simulink model "BugE_v0_40_MAS"  (R2015b)
settings: Solver=FixedStepDiscrete  StartTime=0.0  StopTime=inf  FixedStep=sample_time  RelTol=1e-3
values from neighbouring files (symbols this model uses):
  AB_diode_dV = 0.9    [main_sync.m]
  air_density = 1.225    [main_sync.m]
  bus_charger_Pmax = 1000    [main_sync.m]
  bus_load_Pmax_abs = 500    [main_sync.m]
  capInitVolt = capVmax*sqrt(capInitSoC)    [main_sync.m]
  cyc_kph = [cyc_kph(:,1), cyc_kph(:,2)*speed_max_limit/speed_max]    [main_sync.m]
  cyc_repeat = 0    [main_sync.m]
  ess1_init_soc = 1    [main_sync.m]
  ess1_soh = 1    [main_sync.m]
  ess2_init_soc = 1    [main_sync.m]
  ess2_soh = 1    [main_sync.m]
  ess3_init_soc = 1    [main_sync.m]
  ess3_soh = 1    [main_sync.m]
  ess4_init_soc = 1    [main_sync.m]
  ess4_soh = 1    [main_sync.m]
  ess5_init_soc = 1    [main_sync.m]
  ess5_soh = 1    [main_sync.m]
  gear_ratio = 6    [main_sync.m]
  loadpower = rawcsv(:,2)    [main_sync.m]
  loadtime = rawcsv(:,1)    [main_sync.m]
  lockSOCs = 0    [main_sync.m]
  max_brk_torque = 300    [main_sync.m]
  no_wheels = 3    [main_sync.m]
  period2 = max(loadtime)    [main_sync.m]
  PV_Pmax = 100    [main_sync.m]
  sample_time = 0.01    [main_sync.m]
  startup_seq_step_delay = 0.2    [main_sync.m]
  stop_option = 0    [main_sync.m]
  use_drive_cycle = 1    [main_sync.m]
  use_real_subs_loads = 1    [main_sync.m]
  vbus_max = 25    [main_sync.m]
  vbus_min = 17    [main_sync.m]
  vbus_safety_threshold = 2    [main_sync.m]
  vbus_threshold = 20    [main_sync.m]
  veh_CD = 0.35    [main_sync.m]
  veh_FA = 1.543    [main_sync.m]
  veh_gravity = 9.81*veh_mass    (= 1863.9)    [main_sync.m]
  veh_mass = 190    [main_sync.m]
  wh_1st_rrc = 0.02    [main_sync.m]
  wh_bearing_frc = 0.0015    [main_sync.m]
  wh_inertia = 0.0556    [main_sync.m]
  wh_radius = 0.508/2    (= 0.254)    [main_sync.m]
undefined symbols (not defined in the file or in its folder): capC, capR, cyc_acc, cyc_avg_time_samples, cyc_brk, cyc_grade, cyc_key, DCM_eff_factor_for_Vin, DCM_eff_for_Iout, DCM_Iout, DCM_Iout_max, DCM_Pin_noload, DCM_Pout_max, DCM_Vin, DCM_Vout, DiscIntNeverNeededParam, ess2_coulombic_eff, ess2_Ineg_max_SOC, ess2_Ineg_max_temp, ess2_Ipos_max_SOC, ess2_Ipos_max_temp, ess2_max_ah_cap, ess2_max_volts, ess2_min_volts, ess2_module_parallel, ess2_module_series, ess2_r_dis, ess2_soc, ess2_SOC_for_Ilimit, ess2_temp_for_Ilimit, ess2_temp_max, ess2_tmp, ess2_voc, ess3_coulombic_eff, ess3_max_ah_cap, ess3_module_parallel, ess3_module_series, ess3_r_dis, ess3_soc, ess3_tmp, ess3_voc, ess_coulombic_eff, ess_Ineg_max_SOC, ess_Ineg_max_temp, ess_Ipos_max_SOC, ess_Ipos_max_temp, ess_max_ah_cap, ess_max_volts, ess_min_volts, ess_module_parallel, ess_module_series, ess_nominal_volts, ess_r_dis, ess_soc, ess_SOC_for_Ilimit, ess_temp_for_Ilimit, ess_temp_max, ess_tmp, ess_voc, MC_eff1 ... (+17)
libraries: simulink x139, commfilt2 x1, simulink_extras x1
(part 5 of 7)

== system BugE_v0_40_MAS/Master Controller/Secondary Objectives/Motor MBDCDC boost ==
  enable : Inport
  Bus Selector : BusSelector  OutputSignals=MB_droop
  Product : Product
  Saturation : Saturate  UpperLimit=0  LowerLimit=vbus_min-vbus_max
  Switch1 : Switch  Criteria=u2 > Threshold
  "[0.05, inf)" : DeadZone  LowerValue=-inf  UpperValue=0.05  SaturateOnIntegerOverflow=on
  boost off : Logic  Operator=NOT  AllPortsSameDT=off  OutDataTypeStr=boolean
  d Imotor / d t : simulink/Discrete/Discrete Derivative  gainval=1.0  ICPrevScaledInput=0.0  InputProcessing=Inherited  OutMin=[]  OutMax=[]  OutDataType=fixdt(1, 16)  OutScaling=2^-10  DoSatur=off
  moving average 50ms : DiscreteFir  Coefficients=ones(1,5)/5  SampleTime=sample_time
  normalize 1 / Imax : Gain  Gain=1/mc_max_crrnt
  ones : Subsystem
  shift gain [d_V0/ (d_I/d_t)] : Gain  Gain=-25
  some MB DCDCs are off : Logic  Operator=NAND  Inputs=1  AllPortsSameDT=off  OutDataTypeStr=boolean
  use boost : Logic  Operator=NOR  AllPortsSameDT=off  OutDataTypeStr=boolean
  zero : Constant  Value=0  SampleTime=sample_time
  MB V0 adj : Outport
  wires:
  shift gain [d_V0/ (d_I/d_t)]/1 -> Saturation/1
  moving average 50ms/1 -> normalize 1 / Imax/1
  enable/1 -> boost off/1
  boost off/1 -> use boost/2
  use boost/1 -> Switch1/2
  some MB DCDCs are off/1 -> use boost/1
  Product/1 -> Switch1/1
  zero/1 -> Switch1/3
  ones/1(O) -> Product/2
  normalize 1 / Imax/1 -> d Imotor / d t/1
  [Drive_current_reading] -> moving average 50ms/1
  Switch1/1 -> MB V0 adj/1
  d Imotor / d t/1 -> "[0.05, inf)"/1
  "[0.05, inf)"/1 -> shift gain [d_V0/ (d_I/d_t)]/1
  Saturation/1 -> Product/1
  [active_droop_bus] -> Bus Selector/1
  Bus Selector/1 -> ones/1(I), some MB DCDCs are off/1  "<MB_droop>"

== system BugE_v0_40_MAS/Master Controller/Secondary Objectives/Source prioritization ==
  enable : Inport
  Bias : Bias  Bias=1
  Bus Selector1 : BusSelector  OutputSignals=CHG_droop,MB_droop,SB_droop
  Gain : Gain  Gain=-1
  Gain1 : Gain  Gain=-2
  Product : Product
  Product1 : Product
  and1 : Logic  AllPortsSameDT=off  OutDataTypeStr=boolean
  and2 : Logic  AllPortsSameDT=off  OutDataTypeStr=boolean
  bool2dbl : DataTypeConversion  OutDataTypeStr=double
  bool2dbl1 : DataTypeConversion  OutDataTypeStr=double
  bool2dbl2 : DataTypeConversion  OutDataTypeStr=double
  charging : Logic  Operator=OR  Inputs=1  AllPortsSameDT=off  OutDataTypeStr=boolean
  SB slope adj : Outport
  MB V0 adj : Outport  Port=2
  SB V0 adj : Outport  Port=3
  wires:
  Bus Selector1/3 -> and1/1  "<SB_droop>"
  Bus Selector1/1 -> charging/1  "<CHG_droop>"
  charging/1 -> bool2dbl/1
  [active_droop_bus] -> Bus Selector1/1
  bool2dbl/1 -> Product1/1, Product/1
  Product/1 -> Gain1/1
  Product1/1 -> Gain/1
  Bias/1 -> SB slope adj/1
  and2/1 -> bool2dbl1/1
  bool2dbl2/1 -> Bias/1, Product1/2
  bool2dbl1/1 -> Product/2
  enable/1 -> and2/2, and1/2
  and1/1 -> bool2dbl2/1
  Bus Selector1/2 -> and2/1  "<MB_droop>"
  Gain1/1 -> MB V0 adj/1
  Gain/1 -> SB V0 adj/1

== system BugE_v0_40_MAS/Master Controller/Signal Buffer/(0 device OFF // 1 ON)1 ==
  EN : Inport
  DSBL : Inport  Port=2
  2dbl : DataTypeConversion  OutDataTypeStr=double
  2dbl1 : DataTypeConversion  OutDataTypeStr=double
  Detect Increase : simulink/Logic and Bit Operations/Detect Increase  vinit=0.0  InputProcessing=Inherited  OutDataTypeStr=boolean
  Detect Increase1 : simulink/Logic and Bit Operations/Detect Increase  vinit=0.0  InputProcessing=Inherited  OutDataTypeStr=boolean
  OR : Sum
  Switch : Switch  Criteria=u2 > Threshold
  Switch1 : Switch  Criteria=u2 > Threshold
  Unit Delay : UnitDelay  SampleTime=sample_time
  disable : Constant  Value=0  OutDataTypeStr=boolean  SampleTime=sample_time
  enable : Constant  OutDataTypeStr=boolean  SampleTime=sample_time
  state : Outport
  wires:
  EN/1 -> Detect Increase/1
  Detect Increase1/1 -> 2dbl1/1
  Switch/1 -> state/1, Unit Delay/1
  DSBL/1 -> Detect Increase1/1
  OR/1 -> Switch/2
  Detect Increase/1 -> 2dbl/1
  Unit Delay/1 -> Switch/3
  disable/1 -> Switch1/1
  enable/1 -> Switch1/3
  Switch1/1 -> Switch/1
  2dbl1/1 -> Switch1/2, OR/2
  2dbl/1 -> OR/1

== system BugE_v0_40_MAS/Master Controller/Signal Buffer/(0 device OFF // 1 ON)10 ==
  EN : Inport
  DSBL : Inport  Port=2
  2dbl : DataTypeConversion  OutDataTypeStr=double
  2dbl1 : DataTypeConversion  OutDataTypeStr=double
  Detect Increase : simulink/Logic and Bit Operations/Detect Increase  vinit=0.0  InputProcessing=Inherited  OutDataTypeStr=boolean
  Detect Increase1 : simulink/Logic and Bit Operations/Detect Increase  vinit=0.0  InputProcessing=Inherited  OutDataTypeStr=boolean
  OR : Sum
  Switch : Switch  Criteria=u2 > Threshold
  Switch1 : Switch  Criteria=u2 > Threshold
  Unit Delay : UnitDelay  SampleTime=sample_time
  disable : Constant  Value=0  OutDataTypeStr=boolean  SampleTime=sample_time
  enable : Constant  OutDataTypeStr=boolean  SampleTime=sample_time
  state : Outport
  wires:
  EN/1 -> Detect Increase/1
  Detect Increase1/1 -> 2dbl1/1
  Switch/1 -> state/1, Unit Delay/1
  DSBL/1 -> Detect Increase1/1
  OR/1 -> Switch/2
  Detect Increase/1 -> 2dbl/1
  Unit Delay/1 -> Switch/3
  disable/1 -> Switch1/1
  enable/1 -> Switch1/3
  Switch1/1 -> Switch/1
  2dbl1/1 -> Switch1/2, OR/2
  2dbl/1 -> OR/1

== system BugE_v0_40_MAS/Master Controller/Signal Buffer/(0 device OFF // 1 ON)11 ==
  EN : Inport
  DSBL : Inport  Port=2
  2dbl : DataTypeConversion  OutDataTypeStr=double
  2dbl1 : DataTypeConversion  OutDataTypeStr=double
  Detect Increase : simulink/Logic and Bit Operations/Detect Increase  vinit=0.0  InputProcessing=Inherited  OutDataTypeStr=boolean
  Detect Increase1 : simulink/Logic and Bit Operations/Detect Increase  vinit=0.0  InputProcessing=Inherited  OutDataTypeStr=boolean
  OR : Sum
  Switch : Switch  Criteria=u2 > Threshold
  Switch1 : Switch  Criteria=u2 > Threshold
  Unit Delay : UnitDelay  SampleTime=sample_time
  disable : Constant  Value=0  OutDataTypeStr=boolean  SampleTime=sample_time
  enable : Constant  OutDataTypeStr=boolean  SampleTime=sample_time
  state : Outport
  wires:
  EN/1 -> Detect Increase/1
  Detect Increase1/1 -> 2dbl1/1
  Switch/1 -> state/1, Unit Delay/1
  DSBL/1 -> Detect Increase1/1
  OR/1 -> Switch/2
  Detect Increase/1 -> 2dbl/1
  Unit Delay/1 -> Switch/3
  disable/1 -> Switch1/1
  enable/1 -> Switch1/3
  Switch1/1 -> Switch/1
  2dbl1/1 -> Switch1/2, OR/2
  2dbl/1 -> OR/1

== system BugE_v0_40_MAS/Master Controller/Signal Buffer/(0 device OFF // 1 ON)12 ==
  EN : Inport
  DSBL : Inport  Port=2
  2dbl : DataTypeConversion  OutDataTypeStr=double
  2dbl1 : DataTypeConversion  OutDataTypeStr=double
  Detect Increase : simulink/Logic and Bit Operations/Detect Increase  vinit=0.0  InputProcessing=Inherited  OutDataTypeStr=boolean
  Detect Increase1 : simulink/Logic and Bit Operations/Detect Increase  vinit=0.0  InputProcessing=Inherited  OutDataTypeStr=boolean
  OR : Sum
  Switch : Switch  Criteria=u2 > Threshold
  Switch1 : Switch  Criteria=u2 > Threshold
  Unit Delay : UnitDelay  SampleTime=sample_time
  disable : Constant  Value=0  OutDataTypeStr=boolean  SampleTime=sample_time
  enable : Constant  OutDataTypeStr=boolean  SampleTime=sample_time
  state : Outport
  wires:
  EN/1 -> Detect Increase/1
  Detect Increase1/1 -> 2dbl1/1
  Switch/1 -> state/1, Unit Delay/1
  DSBL/1 -> Detect Increase1/1
  OR/1 -> Switch/2
  Detect Increase/1 -> 2dbl/1
  Unit Delay/1 -> Switch/3
  disable/1 -> Switch1/1
  enable/1 -> Switch1/3
  Switch1/1 -> Switch/1
  2dbl1/1 -> Switch1/2, OR/2
  2dbl/1 -> OR/1

== system BugE_v0_40_MAS/Master Controller/Signal Buffer/(0 device OFF // 1 ON)13 ==
  EN : Inport
  DSBL : Inport  Port=2
  2dbl : DataTypeConversion  OutDataTypeStr=double
  2dbl1 : DataTypeConversion  OutDataTypeStr=double
  Detect Increase : simulink/Logic and Bit Operations/Detect Increase  vinit=0.0  InputProcessing=Inherited  OutDataTypeStr=boolean
  Detect Increase1 : simulink/Logic and Bit Operations/Detect Increase  vinit=0.0  InputProcessing=Inherited  OutDataTypeStr=boolean
  OR : Sum
  Switch : Switch  Criteria=u2 > Threshold
  Switch1 : Switch  Criteria=u2 > Threshold
  Unit Delay : UnitDelay  SampleTime=sample_time
  disable : Constant  Value=0  OutDataTypeStr=boolean  SampleTime=sample_time
  enable : Constant  OutDataTypeStr=boolean  SampleTime=sample_time
  state : Outport
  wires:
  EN/1 -> Detect Increase/1
  Detect Increase1/1 -> 2dbl1/1
  Switch/1 -> state/1, Unit Delay/1
  DSBL/1 -> Detect Increase1/1
  OR/1 -> Switch/2
  Detect Increase/1 -> 2dbl/1
  Unit Delay/1 -> Switch/3
  disable/1 -> Switch1/1
  enable/1 -> Switch1/3
  Switch1/1 -> Switch/1
  2dbl1/1 -> Switch1/2, OR/2
  2dbl/1 -> OR/1

== system BugE_v0_40_MAS/Master Controller/Signal Buffer/(0 device OFF // 1 ON)14 ==
  EN : Inport
  DSBL : Inport  Port=2
  2dbl : DataTypeConversion  OutDataTypeStr=double
  2dbl1 : DataTypeConversion  OutDataTypeStr=double
  Detect Increase : simulink/Logic and Bit Operations/Detect Increase  vinit=0.0  InputProcessing=Inherited  OutDataTypeStr=boolean
  Detect Increase1 : simulink/Logic and Bit Operations/Detect Increase  vinit=0.0  InputProcessing=Inherited  OutDataTypeStr=boolean
  OR : Sum
  Switch : Switch  Criteria=u2 > Threshold
  Switch1 : Switch  Criteria=u2 > Threshold
  Unit Delay : UnitDelay  SampleTime=sample_time
  disable : Constant  Value=0  OutDataTypeStr=boolean  SampleTime=sample_time
  enable : Constant  OutDataTypeStr=boolean  SampleTime=sample_time
  state : Outport
  wires:
  EN/1 -> Detect Increase/1
  Detect Increase1/1 -> 2dbl1/1
  Switch/1 -> state/1, Unit Delay/1
  DSBL/1 -> Detect Increase1/1
  OR/1 -> Switch/2
  Detect Increase/1 -> 2dbl/1
  Unit Delay/1 -> Switch/3
  disable/1 -> Switch1/1
  enable/1 -> Switch1/3
  Switch1/1 -> Switch/1
  2dbl1/1 -> Switch1/2, OR/2
  2dbl/1 -> OR/1

== system BugE_v0_40_MAS/Master Controller/Signal Buffer/(0 device OFF // 1 ON)15 ==
  EN : Inport
  DSBL : Inport  Port=2
  2dbl : DataTypeConversion  OutDataTypeStr=double
  2dbl1 : DataTypeConversion  OutDataTypeStr=double
  Detect Increase : simulink/Logic and Bit Operations/Detect Increase  vinit=0.0  InputProcessing=Inherited  OutDataTypeStr=boolean
  Detect Increase1 : simulink/Logic and Bit Operations/Detect Increase  vinit=0.0  InputProcessing=Inherited  OutDataTypeStr=boolean
  OR : Sum
  Switch : Switch  Criteria=u2 > Threshold
  Switch1 : Switch  Criteria=u2 > Threshold
  Unit Delay : UnitDelay  SampleTime=sample_time
  disable : Constant  Value=0  OutDataTypeStr=boolean  SampleTime=sample_time
  enable : Constant  OutDataTypeStr=boolean  SampleTime=sample_time
  state : Outport
  wires:
  EN/1 -> Detect Increase/1
  Detect Increase1/1 -> 2dbl1/1
  Switch/1 -> state/1, Unit Delay/1
  DSBL/1 -> Detect Increase1/1
  OR/1 -> Switch/2
  Detect Increase/1 -> 2dbl/1
  Unit Delay/1 -> Switch/3
  disable/1 -> Switch1/1
  enable/1 -> Switch1/3
  Switch1/1 -> Switch/1
  2dbl1/1 -> Switch1/2, OR/2
  2dbl/1 -> OR/1

== system BugE_v0_40_MAS/Master Controller/Signal Buffer/(0 device OFF // 1 ON)16 ==
  EN : Inport
  DSBL : Inport  Port=2
  2dbl : DataTypeConversion  OutDataTypeStr=double
  2dbl1 : DataTypeConversion  OutDataTypeStr=double
  Detect Increase : simulink/Logic and Bit Operations/Detect Increase  vinit=0.0  InputProcessing=Inherited  OutDataTypeStr=boolean
  Detect Increase1 : simulink/Logic and Bit Operations/Detect Increase  vinit=0.0  InputProcessing=Inherited  OutDataTypeStr=boolean
  OR : Sum
  Switch : Switch  Criteria=u2 > Threshold
  Switch1 : Switch  Criteria=u2 > Threshold
  Unit Delay : UnitDelay  SampleTime=sample_time
  disable : Constant  Value=0  OutDataTypeStr=boolean  SampleTime=sample_time
  enable : Constant  OutDataTypeStr=boolean  SampleTime=sample_time
  state : Outport
  wires:
  EN/1 -> Detect Increase/1
  Detect Increase1/1 -> 2dbl1/1
  Switch/1 -> state/1, Unit Delay/1
  DSBL/1 -> Detect Increase1/1
  OR/1 -> Switch/2
  Detect Increase/1 -> 2dbl/1
  Unit Delay/1 -> Switch/3
  disable/1 -> Switch1/1
  enable/1 -> Switch1/3
  Switch1/1 -> Switch/1
  2dbl1/1 -> Switch1/2, OR/2
  2dbl/1 -> OR/1

== system BugE_v0_40_MAS/Master Controller/Signal Buffer/(0 device OFF // 1 ON)2 ==
  EN : Inport
  DSBL : Inport  Port=2
  2dbl : DataTypeConversion  OutDataTypeStr=double
  2dbl1 : DataTypeConversion  OutDataTypeStr=double
  Detect Increase : simulink/Logic and Bit Operations/Detect Increase  vinit=0.0  InputProcessing=Inherited  OutDataTypeStr=boolean
  Detect Increase1 : simulink/Logic and Bit Operations/Detect Increase  vinit=0.0  InputProcessing=Inherited  OutDataTypeStr=boolean
  OR : Sum
  Switch : Switch  Criteria=u2 > Threshold
  Switch1 : Switch  Criteria=u2 > Threshold
  Unit Delay : UnitDelay  SampleTime=sample_time
  disable : Constant  Value=0  OutDataTypeStr=boolean  SampleTime=sample_time
  enable : Constant  OutDataTypeStr=boolean  SampleTime=sample_time
  state : Outport
  wires:
  EN/1 -> Detect Increase/1
  Detect Increase1/1 -> 2dbl1/1
  Switch/1 -> state/1, Unit Delay/1
  DSBL/1 -> Detect Increase1/1
  OR/1 -> Switch/2
  Detect Increase/1 -> 2dbl/1
  Unit Delay/1 -> Switch/3
  disable/1 -> Switch1/1
  enable/1 -> Switch1/3
  Switch1/1 -> Switch/1
  2dbl1/1 -> Switch1/2, OR/2
  2dbl/1 -> OR/1

== system BugE_v0_40_MAS/Master Controller/Signal Buffer/(0 device OFF // 1 ON)3 ==
  EN : Inport
  DSBL : Inport  Port=2
  2dbl : DataTypeConversion  OutDataTypeStr=double
  2dbl1 : DataTypeConversion  OutDataTypeStr=double
  Detect Increase : simulink/Logic and Bit Operations/Detect Increase  vinit=0.0  InputProcessing=Inherited  OutDataTypeStr=boolean
  Detect Increase1 : simulink/Logic and Bit Operations/Detect Increase  vinit=0.0  InputProcessing=Inherited  OutDataTypeStr=boolean
  OR : Sum
  Switch : Switch  Criteria=u2 > Threshold
  Switch1 : Switch  Criteria=u2 > Threshold
  Unit Delay : UnitDelay  SampleTime=sample_time
  disable : Constant  Value=0  OutDataTypeStr=boolean  SampleTime=sample_time
  enable : Constant  OutDataTypeStr=boolean  SampleTime=sample_time
  state : Outport
  wires:
  EN/1 -> Detect Increase/1
  Detect Increase1/1 -> 2dbl1/1
  Switch/1 -> state/1, Unit Delay/1
  DSBL/1 -> Detect Increase1/1
  OR/1 -> Switch/2
  Detect Increase/1 -> 2dbl/1
  Unit Delay/1 -> Switch/3
  disable/1 -> Switch1/1
  enable/1 -> Switch1/3
  Switch1/1 -> Switch/1
  2dbl1/1 -> Switch1/2, OR/2
  2dbl/1 -> OR/1

== system BugE_v0_40_MAS/Master Controller/Signal Buffer/(0 device OFF // 1 ON)4 ==
  EN : Inport
  DSBL : Inport  Port=2
  2dbl : DataTypeConversion  OutDataTypeStr=double
  2dbl1 : DataTypeConversion  OutDataTypeStr=double
  Detect Increase : simulink/Logic and Bit Operations/Detect Increase  vinit=0.0  InputProcessing=Inherited  OutDataTypeStr=boolean
  Detect Increase1 : simulink/Logic and Bit Operations/Detect Increase  vinit=0.0  InputProcessing=Inherited  OutDataTypeStr=boolean
  OR : Sum
  Switch : Switch  Criteria=u2 > Threshold
  Switch1 : Switch  Criteria=u2 > Threshold
  Unit Delay : UnitDelay  SampleTime=sample_time
  disable : Constant  Value=0  OutDataTypeStr=boolean  SampleTime=sample_time
  enable : Constant  OutDataTypeStr=boolean  SampleTime=sample_time
  state : Outport
  wires:
  EN/1 -> Detect Increase/1
  Detect Increase1/1 -> 2dbl1/1
  Switch/1 -> state/1, Unit Delay/1
  DSBL/1 -> Detect Increase1/1
  OR/1 -> Switch/2
  Detect Increase/1 -> 2dbl/1
  Unit Delay/1 -> Switch/3
  disable/1 -> Switch1/1
  enable/1 -> Switch1/3
  Switch1/1 -> Switch/1
  2dbl1/1 -> Switch1/2, OR/2
  2dbl/1 -> OR/1

== system BugE_v0_40_MAS/Master Controller/Signal Buffer/(0 device OFF // 1 ON)5 ==
  EN : Inport
  DSBL : Inport  Port=2
  2dbl : DataTypeConversion  OutDataTypeStr=double
  2dbl1 : DataTypeConversion  OutDataTypeStr=double
  Detect Increase : simulink/Logic and Bit Operations/Detect Increase  vinit=0.0  InputProcessing=Inherited  OutDataTypeStr=boolean
  Detect Increase1 : simulink/Logic and Bit Operations/Detect Increase  vinit=0.0  InputProcessing=Inherited  OutDataTypeStr=boolean
  OR : Sum
  Switch : Switch  Criteria=u2 > Threshold
  Switch1 : Switch  Criteria=u2 > Threshold
  Unit Delay : UnitDelay  SampleTime=sample_time
  disable : Constant  Value=0  OutDataTypeStr=boolean  SampleTime=sample_time
  enable : Constant  OutDataTypeStr=boolean  SampleTime=sample_time
  state : Outport
  wires:
  EN/1 -> Detect Increase/1
  Detect Increase1/1 -> 2dbl1/1
  Switch/1 -> state/1, Unit Delay/1
  DSBL/1 -> Detect Increase1/1
  OR/1 -> Switch/2
  Detect Increase/1 -> 2dbl/1
  Unit Delay/1 -> Switch/3
  disable/1 -> Switch1/1
  enable/1 -> Switch1/3
  Switch1/1 -> Switch/1
  2dbl1/1 -> Switch1/2, OR/2
  2dbl/1 -> OR/1

== system BugE_v0_40_MAS/Master Controller/Signal Buffer/(0 device OFF // 1 ON)6 ==
  EN : Inport
  DSBL : Inport  Port=2
  2dbl : DataTypeConversion  OutDataTypeStr=double
  2dbl1 : DataTypeConversion  OutDataTypeStr=double
  Detect Increase : simulink/Logic and Bit Operations/Detect Increase  vinit=0.0  InputProcessing=Inherited  OutDataTypeStr=boolean
  Detect Increase1 : simulink/Logic and Bit Operations/Detect Increase  vinit=0.0  InputProcessing=Inherited  OutDataTypeStr=boolean
  OR : Sum
  Switch : Switch  Criteria=u2 > Threshold
  Switch1 : Switch  Criteria=u2 > Threshold
  Unit Delay : UnitDelay  SampleTime=sample_time
  disable : Constant  Value=0  OutDataTypeStr=boolean  SampleTime=sample_time
  enable : Constant  OutDataTypeStr=boolean  SampleTime=sample_time
  state : Outport
  wires:
  EN/1 -> Detect Increase/1
  Detect Increase1/1 -> 2dbl1/1
  Switch/1 -> state/1, Unit Delay/1
  DSBL/1 -> Detect Increase1/1
  OR/1 -> Switch/2
  Detect Increase/1 -> 2dbl/1
  Unit Delay/1 -> Switch/3
  disable/1 -> Switch1/1
  enable/1 -> Switch1/3
  Switch1/1 -> Switch/1
  2dbl1/1 -> Switch1/2, OR/2
  2dbl/1 -> OR/1

== system BugE_v0_40_MAS/Master Controller/Signal Buffer/(0 device OFF // 1 ON)7 ==
  EN : Inport
  DSBL : Inport  Port=2
  2dbl : DataTypeConversion  OutDataTypeStr=double
  2dbl1 : DataTypeConversion  OutDataTypeStr=double
  Detect Increase : simulink/Logic and Bit Operations/Detect Increase  vinit=0.0  InputProcessing=Inherited  OutDataTypeStr=boolean
  Detect Increase1 : simulink/Logic and Bit Operations/Detect Increase  vinit=0.0  InputProcessing=Inherited  OutDataTypeStr=boolean
  OR : Sum
  Switch : Switch  Criteria=u2 > Threshold
  Switch1 : Switch  Criteria=u2 > Threshold
  Unit Delay : UnitDelay  SampleTime=sample_time
  disable : Constant  Value=0  OutDataTypeStr=boolean  SampleTime=sample_time
  enable : Constant  OutDataTypeStr=boolean  SampleTime=sample_time
  state : Outport
  wires:
  EN/1 -> Detect Increase/1
  Detect Increase1/1 -> 2dbl1/1
  Switch/1 -> state/1, Unit Delay/1
  DSBL/1 -> Detect Increase1/1
  OR/1 -> Switch/2
  Detect Increase/1 -> 2dbl/1
  Unit Delay/1 -> Switch/3
  disable/1 -> Switch1/1
  enable/1 -> Switch1/3
  Switch1/1 -> Switch/1
  2dbl1/1 -> Switch1/2, OR/2
  2dbl/1 -> OR/1

== system BugE_v0_40_MAS/Master Controller/Signal Buffer/(0 device OFF // 1 ON)8 ==
  EN : Inport
  DSBL : Inport  Port=2
  2dbl : DataTypeConversion  OutDataTypeStr=double
  2dbl1 : DataTypeConversion  OutDataTypeStr=double
  Detect Increase : simulink/Logic and Bit Operations/Detect Increase  vinit=0.0  InputProcessing=Inherited  OutDataTypeStr=boolean
  Detect Increase1 : simulink/Logic and Bit Operations/Detect Increase  vinit=0.0  InputProcessing=Inherited  OutDataTypeStr=boolean
  OR : Sum
  Switch : Switch  Criteria=u2 > Threshold
  Switch1 : Switch  Criteria=u2 > Threshold
  Unit Delay : UnitDelay  SampleTime=sample_time
  disable : Constant  Value=0  OutDataTypeStr=boolean  SampleTime=sample_time
  enable : Constant  OutDataTypeStr=boolean  SampleTime=sample_time
  state : Outport
  wires:
  EN/1 -> Detect Increase/1
  Detect Increase1/1 -> 2dbl1/1
  Switch/1 -> state/1, Unit Delay/1
  DSBL/1 -> Detect Increase1/1
  OR/1 -> Switch/2
  Detect Increase/1 -> 2dbl/1
  Unit Delay/1 -> Switch/3
  disable/1 -> Switch1/1
  enable/1 -> Switch1/3
  Switch1/1 -> Switch/1
  2dbl1/1 -> Switch1/2, OR/2
  2dbl/1 -> OR/1

== system BugE_v0_40_MAS/Master Controller/Signal Buffer/(0 device OFF // 1 ON)9 ==
  EN : Inport
  DSBL : Inport  Port=2
  2dbl : DataTypeConversion  OutDataTypeStr=double
  2dbl1 : DataTypeConversion  OutDataTypeStr=double
  Detect Increase : simulink/Logic and Bit Operations/Detect Increase  vinit=0.0  InputProcessing=Inherited  OutDataTypeStr=boolean
  Detect Increase1 : simulink/Logic and Bit Operations/Detect Increase  vinit=0.0  InputProcessing=Inherited  OutDataTypeStr=boolean
  OR : Sum
  Switch : Switch  Criteria=u2 > Threshold
  Switch1 : Switch  Criteria=u2 > Threshold
  Unit Delay : UnitDelay  SampleTime=sample_time
  disable : Constant  Value=0  OutDataTypeStr=boolean  SampleTime=sample_time
  enable : Constant  OutDataTypeStr=boolean  SampleTime=sample_time
  state : Outport
  wires:
  EN/1 -> Detect Increase/1
  Detect Increase1/1 -> 2dbl1/1
  Switch/1 -> state/1, Unit Delay/1
  DSBL/1 -> Detect Increase1/1
  OR/1 -> Switch/2
  Detect Increase/1 -> 2dbl/1
  Unit Delay/1 -> Switch/3
  disable/1 -> Switch1/1
  enable/1 -> Switch1/3
  Switch1/1 -> Switch/1
  2dbl1/1 -> Switch1/2, OR/2
  2dbl/1 -> OR/1

== system BugE_v0_40_MAS/Master Controller/Signal Buffer/RLYs_and_12V_bus ==
  Bus Creator : BusCreator  Inputs=12
  Bus Selector : BusSelector  OutputSignals=RLY_MB_DSBL,RLY_SB_DSBL,RLY_EDLC_DSBL,RLY_AUX_DSBL,RLY_DRV_DSBL,DDC_DSBL
  Bus Selector1 : BusSelector  OutputSignals=RLY_MB_EN,RLY_SB_EN,RLY_EDLC_EN,RLY_AUX_EN,DDC_EN
  Bus Selector2 : BusSelector  OutputSignals=RLY_MB_EN,RLY_SB_EN,RLY_MB_DSBL,RLY_SB_DSBL,RLY_DRV_DSBL
  Bus Selector3 : BusSelector  OutputSignals=RLY_MB_EN,RLY_SB_EN,RLY_MB_DSBL,RLY_SB_DSBL,RLY_DRV_EN
  Gain{,1..6} (7 alike) : Gain  OutDataTypeStr=double
  OR10 : Sum  Inputs=+++  AccumDataTypeStr=double  OutDataTypeStr=double
  OR12 : Sum  OutDataTypeStr=double
  OR7 : Sum  Inputs=+++  OutDataTypeStr=double
  OR8 : Sum  Inputs=+++  OutDataTypeStr=double
  OR9 : Sum  Inputs=+++  OutDataTypeStr=double
  Out1 : Outport
  wires:
  Bus Creator/1 -> Out1/1
  OR10/1 -> Bus Creator/4  "RLY_SB_EN"
  Bus Selector2/2 -> OR10/2  "<RLY_SB_EN>"
  Bus Selector2/5 -> OR12/2  "<RLY_DRV_DSBL>"
  Bus Selector/5 -> OR12/1  "<RLY_DRV_DSBL>"
  OR7/1 -> Bus Creator/1  "RLY_MB_DSBL"
  [RLYs_and_12V_bus3] -> Bus Selector2/1
  Gain5/1 -> Bus Creator/5  "RLY_AUX_DSBL"
  Bus Selector/1 -> OR7/1  "<RLY_MB_DSBL>"
  Bus Selector1/1 -> OR9/1  "<RLY_MB_EN>"
  Gain6/1 -> Bus Creator/7  "RLY_DRV_EN"
  OR9/1 -> Bus Creator/3  "RLY_MB_EN"
  Bus Selector3/2 -> OR10/3  "<RLY_SB_EN>"
  Bus Selector2/4 -> OR8/2  "<RLY_SB_DSBL>"
  Bus Selector1/4 -> Gain3/1  "<RLY_AUX_EN>"
  Bus Selector3/3 -> OR7/3  "<RLY_MB_DSBL>"
  [RLYs_and_12V_bus2] -> Bus Selector1/1
  Bus Selector/4 -> Gain5/1  "<RLY_AUX_DSBL>"
  Bus Selector2/3 -> OR7/2  "<RLY_MB_DSBL>"
  Bus Selector3/4 -> OR8/3  "<RLY_SB_DSBL>"
  Bus Selector3/5 -> Gain6/1  "<RLY_DRV_EN>"
  OR12/1 -> Bus Creator/6  "RLY_DRV_DSBL"
  Bus Selector/6 -> Gain1/1  "<DDC_DSBL>"
  Bus Selector2/1 -> OR9/2  "<RLY_MB_EN>"
  OR8/1 -> Bus Creator/2  "RLY_SB_DSBL"
  Bus Selector1/5 -> Gain4/1  "<DDC_EN>"
  [RLYs_and_12V_bus4] -> Bus Selector3/1
  Bus Selector3/1 -> OR9/3  "<RLY_MB_EN>"
  Bus Selector1/2 -> OR10/1  "<RLY_SB_EN>"
  Bus Selector/3 -> Gain/1  "<RLY_EDLC_DSBL>"
  Bus Selector1/3 -> Gain2/1  "<RLY_EDLC_EN>"
  Bus Selector/2 -> OR8/1  "<RLY_SB_DSBL>"
  [RLYs_and_12V_bus] -> Bus Selector/1
  Gain/1 -> Bus Creator/8  "RLY_EDLC_DSBL"
  Gain1/1 -> Bus Creator/9  "DDC_DSBL"
  Gain2/1 -> Bus Creator/10  "RLY_EDLC_EN"
  Gain3/1 -> Bus Creator/11  "RLY_AUX_EN"
  Gain4/1 -> Bus Creator/12  "DDC_EN"

== system BugE_v0_40_MAS/Master Controller/Signal Buffer/droop_bus ==
  Bus Creator : BusCreator  Inputs=10
  Bus Selector2 : BusSelector  OutputSignals=MB_droop_DSBL,SB_droop_DSBL,FE_droop_DSBL,CHG_droop_DSBL,LD_droop_DSBL
  Bus Selector3 : BusSelector  OutputSignals=MB_droop_EN,SB_droop_EN,FE_droop_EN,CHG_droop_EN,LD_droop_EN
  Bus Selector4 : BusSelector  OutputSignals=MB_droop_EN,SB_droop_EN,FE_droop_EN,CHG_droop_EN,LD_droop_EN,MB_droop_DSBL,SB_droop_DSBL,FE_droop_DSBL,CHG_droop_DSBL,LD_droop_DSBL
  Bus Selector6 : BusSelector  OutputSignals=MB_droop_EN,SB_droop_EN,FE_droop_EN,CHG_droop_EN,LD_droop_EN,MB_droop_DSBL,SB_droop_DSBL,FE_droop_DSBL,CHG_droop_DSBL,LD_droop_DSBL
  OR{1..7,12,14,16} (10 alike) : Sum  Inputs=+++  OutDataTypeStr=double
  Out1 : Outport
  wires:
  OR3/1 -> Bus Creator/4  "SB_droop_EN"
  OR1/1 -> Bus Creator/2  "MB_droop_EN"
  OR4/1 -> Bus Creator/5  "FE_droop_DSBL"
  OR2/1 -> Bus Creator/3  "SB_droop_DSBL"
  OR12/1 -> Bus Creator/6  "FE_droop_EN"
  [droop_bus] -> Bus Selector2/1
  Bus Selector4/7 -> OR2/2  "<SB_droop_DSBL>"
  Bus Selector2/4 -> OR5/1  "<CHG_droop_DSBL>"
  [droop_bus2] -> Bus Selector3/1
  Bus Selector4/10 -> OR6/2  "<LD_droop_DSBL>"
  [droop_bus3] -> Bus Selector4/1
  Bus Selector3/4 -> OR14/1  "<CHG_droop_EN>"
  Bus Selector4/4 -> OR14/2  "<CHG_droop_EN>"
  Bus Selector3/3 -> OR12/1  "<FE_droop_EN>"
  Bus Selector4/6 -> OR7/2  "<MB_droop_DSBL>"
  Bus Selector2/1 -> OR7/1  "<MB_droop_DSBL>"
  Bus Selector4/2 -> OR3/2  "<SB_droop_EN>"
  Bus Selector3/1 -> OR1/1  "<MB_droop_EN>"
  Bus Creator/1 -> Out1/1
  OR16/1 -> Bus Creator/10  "LD_droop_EN"
  OR6/1 -> Bus Creator/9  "LD_droop_DSBL"
  Bus Selector4/9 -> OR5/2  "<CHG_droop_DSBL>"
  Bus Selector6/6 -> OR7/3  "<MB_droop_DSBL>"
  Bus Selector6/8 -> OR4/3  "<FE_droop_DSBL>"
  Bus Selector6/4 -> OR14/3  "<CHG_droop_EN>"
  OR14/1 -> Bus Creator/8  "CHG_droop_EN"
  Bus Selector4/3 -> OR12/2  "<FE_droop_EN>"
  Bus Selector4/1 -> OR1/2  "<MB_droop_EN>"
  OR5/1 -> Bus Creator/7  "CHG_droop_DSBL"
  Bus Selector6/7 -> OR2/3  "<SB_droop_DSBL>"
  Bus Selector3/2 -> OR3/1  "<SB_droop_EN>"
  Bus Selector3/5 -> OR16/1  "<LD_droop_EN>"
  Bus Selector2/2 -> OR2/1  "<SB_droop_DSBL>"
  Bus Selector6/3 -> OR12/3  "<FE_droop_EN>"
  Bus Selector2/3 -> OR4/1  "<FE_droop_DSBL>"
  Bus Selector6/10 -> OR6/3  "<LD_droop_DSBL>"
  [droop_bus4] -> Bus Selector6/1
  Bus Selector6/2 -> OR3/3  "<SB_droop_EN>"
  Bus Selector2/5 -> OR6/1  "<LD_droop_DSBL>"
  Bus Selector4/8 -> OR4/2  "<FE_droop_DSBL>"
  OR7/1 -> Bus Creator/1  "MB_droop_DSBL"
  Bus Selector6/9 -> OR5/3  "<CHG_droop_DSBL>"
  Bus Selector6/5 -> OR16/3  "<LD_droop_EN>"
  Bus Selector6/1 -> OR1/3  "<MB_droop_EN>"
  Bus Selector4/5 -> OR16/2  "<LD_droop_EN>"

== system BugE_v0_40_MAS/Master Controller/Signal Buffer/module_PWR_bus ==
  Bus Creator : BusCreator  Inputs=10
  Bus Selector : BusSelector  OutputSignals=MB_MOD_PWR_DSBL,SB_MOD_PWR_DSBL,FE_PWR_DSBL,CHG_PWR_DSBL,LD_PWR_DSBL
  Bus Selector1 : BusSelector  OutputSignals=MB_PWR_DSBL,SB_PWR_DSBL,FE_PWR_DSBL,CHG_PWR_DSBL,LD_PWR_DSBL,MB_MOD_PWR_EN,SB_MOD_PWR_EN,FE_PWR_EN,CHG_PWR_EN,LD_PWR_EN
  Gain{,1..4} (5 alike) : Gain  OutDataTypeStr=double
  OR{7..8,11,13} (4 alike) : Sum  OutDataTypeStr=double
  OR12 : Sum  AccumDataTypeStr=double  OutDataTypeStr=double
  Out1 : Outport
  wires:
  Bus Creator/1 -> Out1/1
  OR7/1 -> Bus Creator/1  "MB_MOD_PWR_DSBL"
  OR8/1 -> Bus Creator/2  "SB_MOD_PWR_DSBL"
  OR13/1 -> Bus Creator/6  "CHG_PWR_DSBL"
  OR12/1 -> Bus Creator/5  "FE_PWR_DSBL"
  Gain3/1 -> Bus Creator/4  "SB_MOD_PWR_EN"
  OR11/1 -> Bus Creator/7  "LD_PWR_DSBL"
  Gain4/1 -> Bus Creator/3  "MB_MOD_PWR_EN"
  Bus Selector/3 -> OR12/1  "<FE_PWR_DSBL>"
  Bus Selector1/6 -> Gain4/1  "<MB_MOD_PWR_EN>"
  Bus Selector/4 -> OR13/1  "<CHG_PWR_DSBL>"
  Bus Selector/1 -> OR7/1  "<MB_MOD_PWR_DSBL>"
  Bus Selector/2 -> OR8/1  "<SB_MOD_PWR_DSBL>"
  Bus Selector1/9 -> Gain1/1  "<CHG_PWR_EN>"
  Bus Selector1/7 -> Gain3/1  "<SB_MOD_PWR_EN>"
  Bus Selector1/10 -> Gain2/1  "<LD_PWR_EN>"
  Bus Selector1/8 -> Gain/1  "<FE_PWR_EN>"
  Bus Selector/5 -> OR11/1  "<LD_PWR_DSBL>"
  [module_PWR_bus2] -> Bus Selector1/1
  [module_PWR_bus] -> Bus Selector/1
  Gain/1 -> Bus Creator/8  "FE_PWR_EN"
  Gain1/1 -> Bus Creator/9  "CHG_PWR_EN"
  Gain2/1 -> Bus Creator/10  "LD_PWR_EN"
  Bus Selector1/1 -> OR7/2  "<MB_PWR_DSBL>"
  Bus Selector1/2 -> OR8/2  "<SB_PWR_DSBL>"
  Bus Selector1/3 -> OR12/2  "<FE_PWR_DSBL>"
  Bus Selector1/4 -> OR13/2  "<CHG_PWR_DSBL>"
  Bus Selector1/5 -> OR11/2  "<LD_PWR_DSBL>"

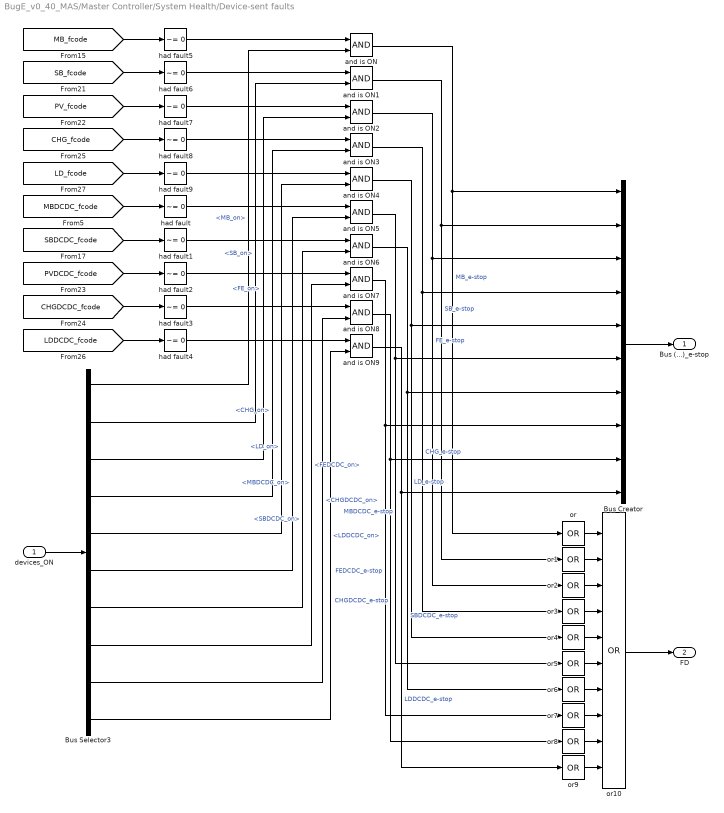
== system BugE_v0_40_MAS/Master Controller/System Health/Device-sent faults ==
  devices_ON : Inport
  Bus Creator : BusCreator  Inputs=10
  Bus Selector3 : BusSelector  OutputSignals=MB_on,SB_on,FE_on,CHG_on,LD_on,MBDCDC_on,SBDCDC_on,FEDCDC_on,CHGDCDC_on,LDDCDC_on
  and is ON{,1..9} (10 alike) : Logic  AllPortsSameDT=off  OutDataTypeStr=boolean
  had fault{,1..9} (10 alike) : simulink/Logic and Bit Operations/Compare To Constant  relop=~=  const=0  OutDataTypeStr=boolean
  or{,1..9} (10 alike) : Logic  Operator=OR  Inputs=1  AllPortsSameDT=off  OutDataTypeStr=boolean
  or10 : Logic  Operator=OR  Inputs=10  AllPortsSameDT=off  OutDataTypeStr=boolean
  Bus (...)_e-stop : Outport
  FD : Outport  Port=2
  wires:
  [MB_fcode] -> had fault5/1
  [SB_fcode] -> had fault6/1
  and is ON4/1 -> or4/1, Bus Creator/5  "LD_e-stop"
  and is ON2/1 -> or2/1, Bus Creator/3  "FE_e-stop"
  [PV_fcode] -> had fault7/1
  and is ON1/1 -> or1/1, Bus Creator/2  "SB_e-stop"
  and is ON3/1 -> or3/1, Bus Creator/4  "CHG_e-stop"
  and is ON/1 -> Bus Creator/1, or/1  "MB_e-stop"
  [CHG_fcode] -> had fault8/1
  [LD_fcode] -> had fault9/1
  and is ON5/1 -> Bus Creator/6, or5/1  "MBDCDC_e-stop"
  and is ON6/1 -> Bus Creator/7, or6/1  "SBDCDC_e-stop"
  and is ON7/1 -> or7/1, Bus Creator/8  "FEDCDC_e-stop"
  and is ON8/1 -> or8/1, Bus Creator/9  "CHGDCDC_e-stop"
  and is ON9/1 -> or9/1, Bus Creator/10  "LDDCDC_e-stop"
  Bus Creator/1 -> Bus (...)_e-stop/1
  or/1 -> or10/1
  or1/1 -> or10/2
  or2/1 -> or10/3
  or3/1 -> or10/4
  or4/1 -> or10/5
  or5/1 -> or10/6
  or6/1 -> or10/7
  or7/1 -> or10/8
  or8/1 -> or10/9
  or9/1 -> or10/10
  or10/1 -> FD/1
  devices_ON/1 -> Bus Selector3/1
  had fault5/1 -> and is ON/1
  had fault6/1 -> and is ON1/1
  had fault7/1 -> and is ON2/1
  had fault8/1 -> and is ON3/1
  had fault9/1 -> and is ON4/1
  had fault/1 -> and is ON5/1
  had fault1/1 -> and is ON6/1
  had fault2/1 -> and is ON7/1
  had fault3/1 -> and is ON8/1
  had fault4/1 -> and is ON9/1
  Bus Selector3/1 -> and is ON/2  "<MB_on>"
  Bus Selector3/2 -> and is ON1/2  "<SB_on>"
  Bus Selector3/3 -> and is ON2/2  "<FE_on>"
  Bus Selector3/4 -> and is ON3/2  "<CHG_on>"
  Bus Selector3/5 -> and is ON4/2  "<LD_on>"
  Bus Selector3/6 -> and is ON5/2  "<MBDCDC_on>"
  Bus Selector3/7 -> and is ON6/2  "<SBDCDC_on>"
  Bus Selector3/9 -> and is ON8/2  "<CHGDCDC_on>"
  Bus Selector3/8 -> and is ON7/2  "<FEDCDC_on>"
  Bus Selector3/10 -> and is ON9/2  "<LDDCDC_on>"
  [MBDCDC_fcode] -> had fault/1
  [SBDCDC_fcode] -> had fault1/1
  [PVDCDC_fcode] -> had fault2/1
  [CHGDCDC_fcode] -> had fault3/1
  [LDDCDC_fcode] -> had fault4/1
